simulink model "x25_CPM_130_Causal"  (R2024b)
settings: Solver=VariableStepAuto  StartTime=0.0  StopTime=3  RelTol=1e-3
InitFcn:
  | run("parametres.m")
  | %data = lire_csv_rc4("Echelon_CH_P50_HG.csv")
values from neighbouring files (symbols this model uses):
  fv = 2.e-6    (= 2e-06)    [parametres.m]
  ISAT = 1.2    [parametres.m]
  Jm = Jm+Jr    (= 1.6219e-06)    [parametres.m]
  Kadapt = Kcapt/r/pas    (= 6382.27146814)    [parametres.m]
  Kcapt = 512*4/2/pi    (= 325.949323452)    [parametres.m]
  Kcm = 25.6e-3    (= 0.0256)    [parametres.m]
  KCou_I = 1000    [parametres.m]
  KCou_P = 1000    [parametres.m]
  KDSI = KPos_D*80/1000000    (= 0.0144)    [parametres.m]
  Kem = 1/(373 *2*pi/60)    (= 0.0256013313285)    [parametres.m]
  KPos_I = 500    [parametres.m]
  KPos_P = 130    [parametres.m]
  KPSI = KPos_P*10/1000    (= 1.3)    [parametres.m]
  Lm = 0.278e-3    (= 0.000278)    [parametres.m]
  pas = 5 /2/pi    (= 0.795774715459)    [parametres.m]
  r = 361/5625    (= 0.0641777777778)    [parametres.m]
  Rm = 2.14    [parametres.m]
  Unom = 24    [parametres.m]
libraries: simulink x2
settings Model: Creator=xavier.pessoles2  LastModifiedBy=xpess

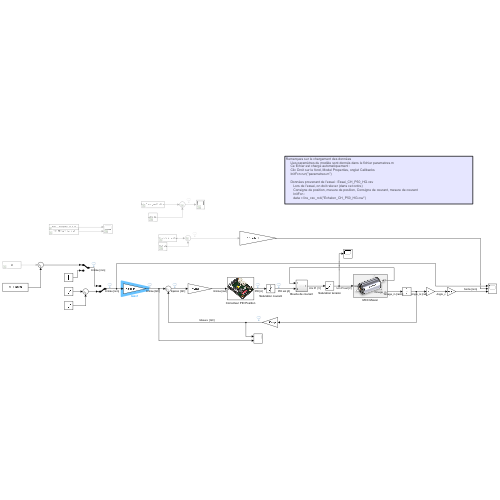
[thumbnail: Simulink's stored preview of the top-level diagram]
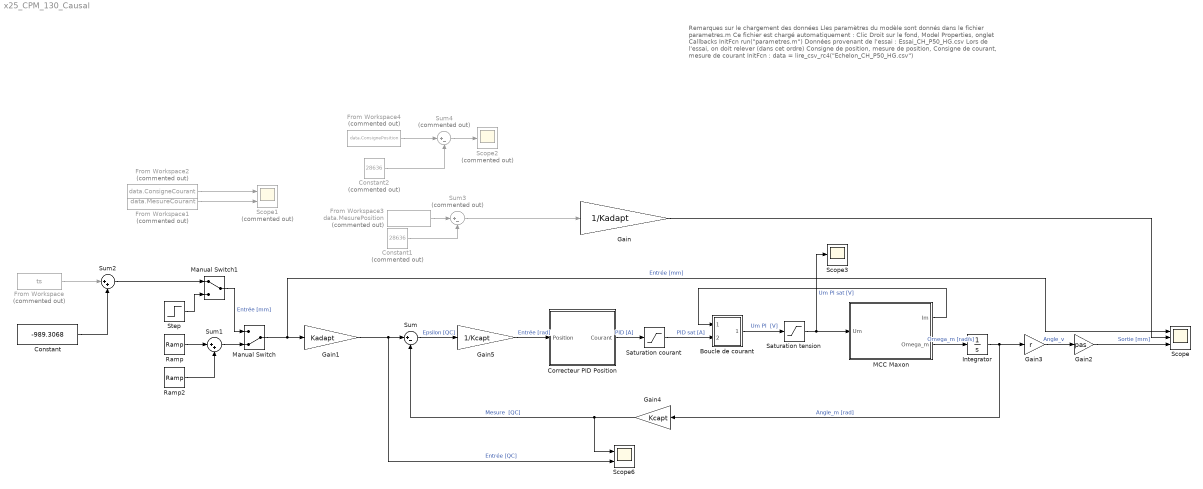
== system x25_CPM_130_Causal ==
  note: Remarques sur le chargement des données
      |      Lles paramètres du modèle sont donnés dans le fichier parametres.m
      |      Ce fichier est chargé automatiquement :
      |      Clic Droit sur le fond, Model Properties, onglet Callbacks
      |      InitFcn run("parametres.m")
      |
      |      Données provenant de l'essai : Essai_CH_P50_HG.csv
      |         Lors de l'essai, on doit relever (dans cet ordre)
      |         Consigne de position, mesure de position, Consigne de courant, mesure de courant
      |         InitFcn :
      |         data = lire_csv_rc4("Echelon_CH_P50_HG.csv")
  Boucle de courant : Subsystem
  Constant : Constant  Value=-989.3068
  Constant1 : Constant  Commented=on  Value=28636
  Constant2 : Constant  Commented=on  Value=28636
  Correcteur PID Position : Subsystem
      mask Display: image('EPOS.png');
  From Workspace : FromWorkspace  Commented=on  VariableName=ts
  From Workspace1 : FromWorkspace  Commented=on  VariableName=data.MesureCourant  SampleTime=0.01
  From Workspace2 : FromWorkspace  Commented=on  VariableName=data.ConsigneCourant  SampleTime=0.01
  From Workspace3 : FromWorkspace  Commented=on  VariableName=data.MesurePosition  SampleTime=0.01
  From Workspace4 : FromWorkspace  Commented=on  VariableName=data.ConsignePosition  SampleTime=0.01
  Gain : Gain  Gain=1/Kadapt
  Gain1 : Gain  Gain=Kadapt
  Gain2 : Gain  Gain=pas
  Gain3 : Gain  Gain=r
  Gain4 : Gain  Gain=Kcapt
  Gain5 : Gain  Gain=1/Kcapt
  Integrator : Integrator
  MCC Maxon : Subsystem
      mask Display: image('MCC.png');
  Manual Switch : ManualSwitch  CurrentSetting=0
  Manual Switch1 : ManualSwitch
  Ramp : simulink/Sources/Ramp  slope=58.14  start=0  InitialOutput=0
  Ramp2 : simulink/Sources/Ramp  slope=-58.14  start=0.86  InitialOutput=0
  Saturation courant : Saturate  UpperLimit=ISAT*1000  LowerLimit=-ISAT*1000
  Saturation tension : Saturate  UpperLimit=Unom  LowerLimit=-Unom
  Scope : Scope  NumInputPorts=3
  Scope1 : Scope  Commented=on  NumInputPorts=2
  Scope2 : Scope  Commented=on
  Scope3 : Scope
  Scope6 : Scope  NumInputPorts=2
  Step : Step  Time=.08  SampleTime=0
  Sum : Sum  Inputs=|+-
  Sum1 : Sum  Inputs=|++
  Sum2 : Sum  Inputs=|++
  Sum3 : Sum  Commented=on  Inputs=|+-
  Sum4 : Sum  Commented=on  Inputs=|+-
  wires:
  MCC Maxon/2(Omega_m) -> Integrator/1  "Omega_m [rad/s]"
  Sum/1 -> Gain5/1  "Epsilon [QC]"
  MCC Maxon/1(Im) -> Boucle de courant/1(In1)
  Correcteur PID Position/1(Courant) -> Saturation courant/1  "PID [A]"
  Boucle de courant/1(Out1) -> Saturation tension/1  "Um PI  [V]"
  Gain4/1 -> Scope6/1, Sum/2  "Mesure  [QC]"
  Gain1/1 -> Sum/1, Scope6/2  "Entrée [QC]"
  Gain2/1 -> Scope/3  "Sortie [mm]"
  Saturation tension/1 -> MCC Maxon/1(Um), Scope3/1  "Um PI sat [V]"
  Saturation courant/1 -> Boucle de courant/2(In2)  "PID sat [A]"
  Ramp/1 -> Sum1/1
  Ramp2/1 -> Sum1/2
  Sum1/1 -> Manual Switch/2
  Manual Switch/1 -> Gain1/1, Scope/1  "Entrée [mm]"
  Gain5/1 -> Correcteur PID Position/1(Position)  "Entrée [rad]"
  Manual Switch1/1 -> Manual Switch/1  "Entrée [mm]"
  Step/1 -> Manual Switch1/2
  From Workspace/1 -> Sum2/1
  Sum2/1 -> Manual Switch1/1
  Constant/1 -> Sum2/2
  From Workspace1/1 -> Scope1/2
  From Workspace2/1 -> Scope1/1
  From Workspace4/1 -> Sum4/1
  Gain/1 -> Scope/2
  From Workspace3/1 -> Sum3/1
  Sum3/1 -> Gain/1
  Constant1/1 -> Sum3/2
  Constant2/1 -> Sum4/2
  Sum4/1 -> Scope2/1
  Integrator/1 -> Gain4/1, Gain3/1  "Angle_m [rad]"
  Gain3/1 -> Gain2/1  "Angle_v"

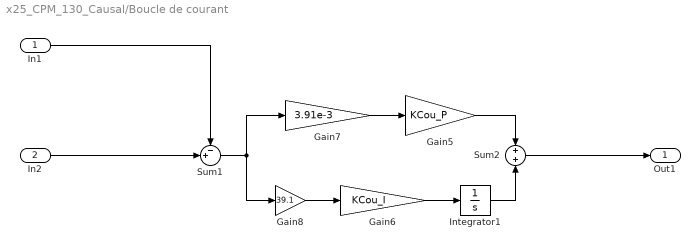
== system x25_CPM_130_Causal/Boucle de courant ==
  In1 : Inport
  In2 : Inport  Port=2
  Gain5 : Gain  Gain=KCou_P
  Gain6 : Gain  Gain=KCou_I
  Gain7 : Gain  Gain=3.91e-3
  Gain8 : Gain  Gain=39.1
  Integrator1 : Integrator
  Sum1 : Sum  Inputs=-+|
  Sum2 : Sum  Inputs=+|+
  Out1 : Outport
  wires:
  Sum1/1 -> Gain7/1, Gain8/1
  Gain5/1 -> Sum2/1
  Sum2/1 -> Out1/1
  Integrator1/1 -> Sum2/2
  Gain8/1 -> Gain6/1
  In1/1 -> Sum1/1
  Gain7/1 -> Gain5/1
  Gain6/1 -> Integrator1/1
  In2/1 -> Sum1/2

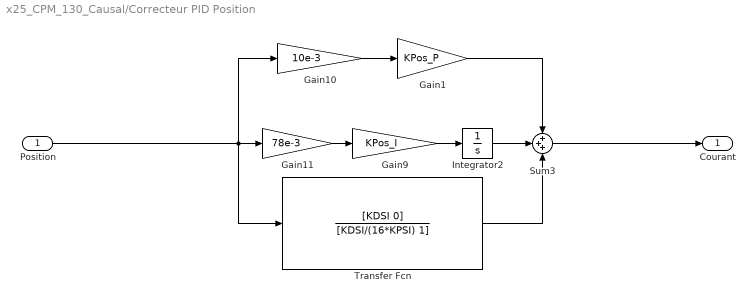
== system x25_CPM_130_Causal/Correcteur PID Position ==
  Position : Inport
  Gain1 : Gain  Gain=KPos_P
  Gain10 : Gain  Gain=10e-3
  Gain11 : Gain  Gain=78e-3
  Gain9 : Gain  Gain=KPos_I
  Integrator2 : Integrator
  Sum3 : Sum  Inputs=+++
  Transfer Fcn : TransferFcn  Numerator=[KDSI 0]  Denominator=[KDSI/(16*KPSI) 1]
  Courant : Outport
  wires:
  Gain1/1 -> Sum3/1
  Position/1 -> Gain10/1, Transfer Fcn/1, Gain11/1
  Gain9/1 -> Integrator2/1
  Sum3/1 -> Courant/1
  Integrator2/1 -> Sum3/2
  Gain10/1 -> Gain1/1
  Gain11/1 -> Gain9/1
  Transfer Fcn/1 -> Sum3/3

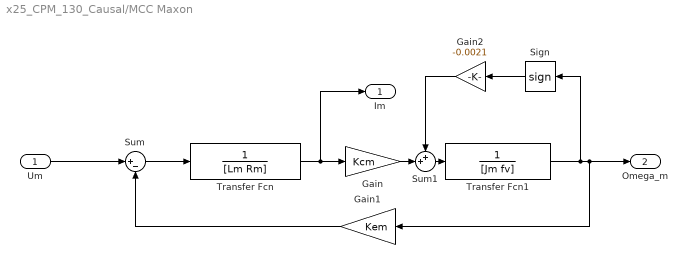
== system x25_CPM_130_Causal/MCC Maxon ==
  Um : Inport
  Gain : Gain  Gain=Kcm
  Gain1 : Gain  Gain=Kem
  Gain2 : Gain  Gain=-0.0021
  Sign : Signum  ZeroCross=off
  Sum : Sum  Inputs=|+-
  Sum1 : Sum  Inputs=++|
  Transfer Fcn : TransferFcn  Denominator=[Lm Rm]
  Transfer Fcn1 : TransferFcn  Denominator=[Jm fv]
  Im : Outport
  Omega_m : Outport  Port=2
  wires:
  Transfer Fcn/1 -> Im/1, Gain/1
  Transfer Fcn1/1 -> Sign/1, Omega_m/1, Gain1/1
  Gain1/1 -> Sum/2
  Um/1 -> Sum/1
  Sum/1 -> Transfer Fcn/1
  Gain/1 -> Sum1/2
  Sum1/1 -> Transfer Fcn1/1
  Sign/1 -> Gain2/1
  Gain2/1 -> Sum1/1
